simulink model "feedback_gravity_comp"  (R2019b)
settings: Solver=FixedStepAuto  StartTime=0.0  StopTime=inf  FixedStep=st  RelTol=1e-3
values from neighbouring files (symbols this model uses):
  p = pi    (= 3.14159265359)    [nominal_model.m]
libraries: arduinolib x18
settings Model: SILPILModeSetting=veronly  ExtModeTrigDuration=2  Creator=paniz  LastModifiedBy=paniz
settings OptimizationCC: EnhancedBackFolding=on  PassReuseOutputArgsAs=Individual arguments  ZeroExternalMemoryAtStartup=off  ZeroInternalMemoryAtStartup=off  MaxStackSize=64  OptimizeBlockOrder=speed  DifferentSizesBufferReuse=on  OptimizationCustomize=off  EfficientTunableParamExpr=on
settings DebuggingCC: ParameterTunabilityLossMsg=error  UnconnectedInputMsg=none  UnconnectedOutputMsg=none  UnconnectedLineMsg=none  SFMachineParentedDataDiag=error
settings HardwareCC: ProdBitPerInt=16  ProdBitPerPointer=16  ProdBitPerSizeT=16  ProdBitPerPtrDiffT=16  ProdLargestAtomicFloat=None  ProdWordSize=8  ProdHWDeviceType=Atmel->AVR
settings SFSimCC: MATLABDynamicMemAlloc=off
settings RTWCC: SystemTargetFile=ert.tlc  HardwareBoard=Arduino Mega 2560  TemplateMakefile=ert_default_tmf  Toolchain=Arduino AVR
settings CodeAppCC: ForceParamTrailComments=on  IgnoreCustomStorageClasses=off  OperatorAnnotations=on  SimulinkDataObjDesc=on  SFDataObjDesc=on  InsertBlockDesc=on
settings ERTTargetCC: SupportContinuousTime=on  SupportVariableSizeSignals=on  ExtMode=on  ExtModeTransport=3  ExtModeStaticAlloc=on  ExtModeStaticAllocSize=2048  ExtModeMexFile=ext_xcp  ExtModeMexArgs=0 5 921600 'C:\Users\paniz\myCodes\Using Arduino and Matlab\Codes\Simulink\3 Muscle with pressure regulator\untitled.elf' 3 1000  ExtModeIntrfLevel=Level2 - Open

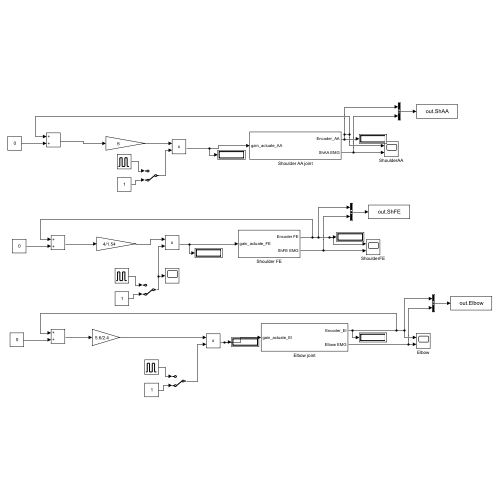
[thumbnail: Simulink's stored preview of the top-level diagram]
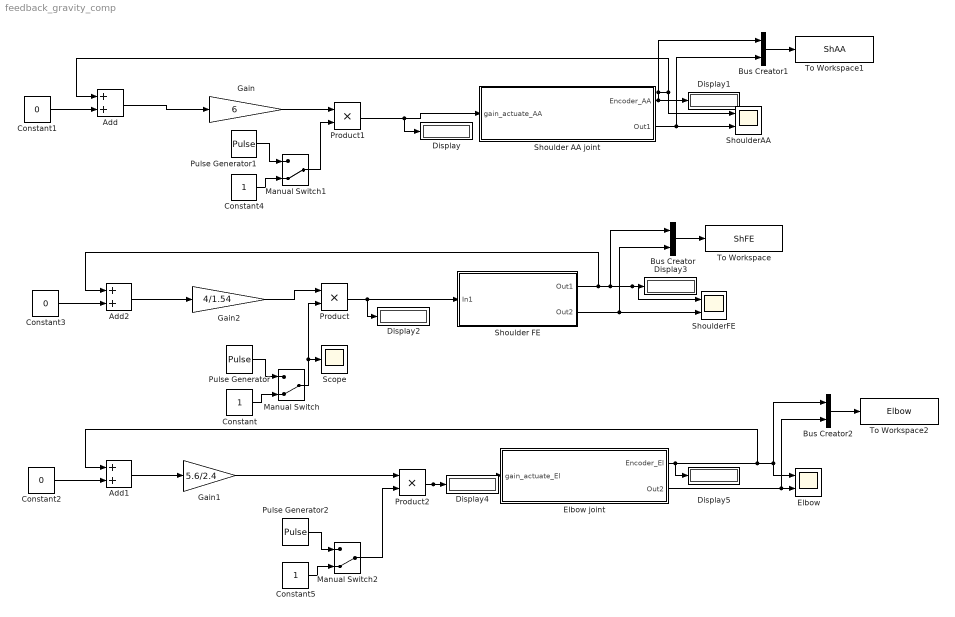
== system feedback_gravity_comp ==
  Add : Sum
  Add1 : Sum
  Add2 : Sum
  Bus Creator : BusCreator  Inputs=2
  Bus Creator1 : BusCreator  Inputs=2
  Bus Creator2 : BusCreator  Inputs=2
  Constant : Constant
  Constant1 : Constant  Value=0
  Constant2 : Constant  Value=0
  Constant3 : Constant  Value=0
  Constant4 : Constant
  Constant5 : Constant
  Display{,1..5} (6 alike) : Display
  Elbow : Scope  NumInputPorts=2
  Elbow joint : Subsystem
  Gain : Gain  Gain=6
  Gain1 : Gain  Gain=5.6/2.4
  Gain2 : Gain  Gain=4/1.54
  Manual Switch : ManualSwitch  CurrentSetting=0
  Manual Switch1 : ManualSwitch  CurrentSetting=0
  Manual Switch2 : ManualSwitch  CurrentSetting=0
  Product : Product
  Product1 : Product
  Product2 : Product
  Pulse Generator : DiscretePulseGenerator  PulseType=Time based  Period=7  PulseWidth=90
  Pulse Generator1 : DiscretePulseGenerator  PulseType=Time based  Period=7  PulseWidth=90
  Pulse Generator2 : DiscretePulseGenerator  PulseType=Time based  Period=7  PulseWidth=90
  Scope : Scope
  Shoulder AA joint : Subsystem
  Shoulder FE : Subsystem
  ShoulderAA : Scope  NumInputPorts=2
  ShoulderFE : Scope  NumInputPorts=2
  To Workspace : ToWorkspace  VariableName=ShFE  SampleTime=-1
  To Workspace1 : ToWorkspace  VariableName=ShAA  SampleTime=-1
  To Workspace2 : ToWorkspace  VariableName=Elbow  SampleTime=-1
  wires:
  Add/1 -> Gain/1
  Constant1/1 -> Add/2
  Constant2/1 -> Add1/2
  Add1/1 -> Gain1/1
  Shoulder AA joint/2(Out1) -> Bus Creator1/2, ShoulderAA/2
  Shoulder AA joint/1(Encoder_AA) -> Bus Creator1/1, ShoulderAA/1, Add/1, Display1/1
  Bus Creator1/1 -> To Workspace1/1
  Elbow joint/2(Out2) -> Bus Creator2/2, Elbow/2
  Elbow joint/1(Encoder_El) -> Elbow/1, Bus Creator2/1, Add1/1, Display5/1
  Bus Creator2/1 -> To Workspace2/1
  Manual Switch1/1 -> Product1/2
  Gain/1 -> Product1/1
  Product1/1 -> Display/1, Shoulder AA joint/1(gain_actuate_AA)
  Manual Switch2/1 -> Product2/2
  Gain1/1 -> Product2/1
  Constant4/1 -> Manual Switch1/2
  Pulse Generator1/1 -> Manual Switch1/1
  Constant5/1 -> Manual Switch2/2
  Pulse Generator2/1 -> Manual Switch2/1
  Manual Switch/1 -> Scope/1, Product/2
  Constant/1 -> Manual Switch/2
  Pulse Generator/1 -> Manual Switch/1
  Gain2/1 -> Product/1
  Product/1 -> Display2/1, Shoulder FE/1(In1)
  Shoulder FE/2(Out2) -> Bus Creator/2, ShoulderFE/2
  Add2/1 -> Gain2/1
  Constant3/1 -> Add2/2
  Shoulder FE/1(Out1) -> Add2/1, Bus Creator/1, ShoulderFE/1, Display3/1
  Bus Creator/1 -> To Workspace/1
  Product2/1 -> Elbow joint/1(gain_actuate_El), Display4/1

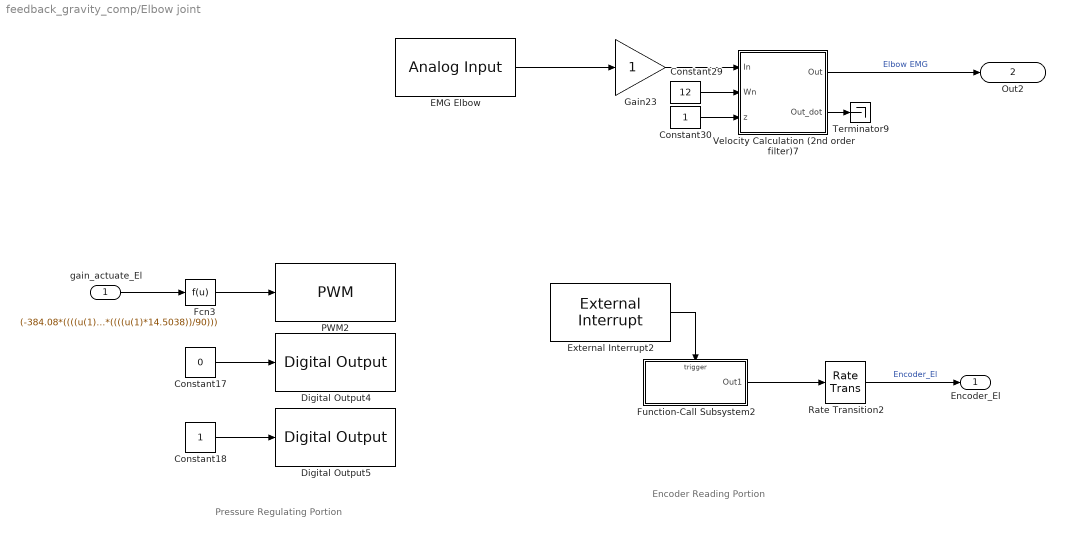
== system feedback_gravity_comp/Elbow joint ==
  note: Pressure Regulating Portion
  note: Encoder Reading Portion
  gain_actuate_El : Inport
  Constant17 : Constant  Value=0  SampleTime=-1
  Constant18 : Constant  SampleTime=-1
  Constant29 : Constant  Value=12
  Constant30 : Constant
  Digital Output4 : arduinolib/Digital Output  pinNumber=17  Direction=output  blockPlatform=arduino
  Digital Output5 : arduinolib/Digital Output  pinNumber=5  Direction=output  blockPlatform=arduino
  EMG Elbow : arduinolib/Analog Input  pinNumber=1  ReadResultsOnly=off  ConversionTriggerSource=Software  ExternalTriggerType=uint32( 0 )  OutputDataType=uint16  EnableConversionCompleteNotify=off  EnableOuputStatus=off  SampleTime=-1  blockPlatform=arduino
  External Interrupt2 : arduinolib/External Interrupt  Pin=3  PullUp=off  Mode=RISING  InterruptSimulationInput=off
      settings: SourceProductBaseCode=ARDUINO
  Fcn3 : Fcn  Expr=(-384.08*((((u(1)*14.5038))/90))^4 + 789.52*((((u(1)*14.5038))/90))^3 - 618.81*((((u(1)*14.5038))/90))^2 + 468.18*((((u(1)*14.5038))/90)))
  Function-Call Subsystem2 : Subsystem  TreatAsAtomicUnit=on
  Gain23 : Gain  OutDataTypeStr=double
  PWM2 : arduinolib/PWM  pinNumber=6  frequencyType=Specify  desiredFrequency=3921.16  achievableFrequency=3921.5686
  Rate Transition2 : RateTransition  Deterministic=off  OutPortSampleTimeOpt=Inherit
  Terminator9 : Terminator
  Velocity Calculation (2nd order filter)7 : Subsystem
  Encoder_El : Outport
  Out2 : Outport  Port=2
  wires:
  gain_actuate_El/1 -> Fcn3/1
  Fcn3/1 -> PWM2/1
  External Interrupt2/1 -> Function-Call Subsystem2/Trigger
  Function-Call Subsystem2/1(Out1) -> Rate Transition2/1
  Constant18/1 -> Digital Output5/1
  Constant17/1 -> Digital Output4/1
  Rate Transition2/1 -> Encoder_El/1  "Encoder_El"
  Velocity Calculation (2nd order filter)7/2(Out_dot) -> Terminator9/1
  EMG Elbow/1 -> Gain23/1
  Constant29/1 -> Velocity Calculation (2nd order filter)7/2(Wn)
  Gain23/1 -> Velocity Calculation (2nd order filter)7/1(In)
  Constant30/1 -> Velocity Calculation (2nd order filter)7/3(z)
  Velocity Calculation (2nd order filter)7/1(Out) -> Out2/1  "Elbow EMG"

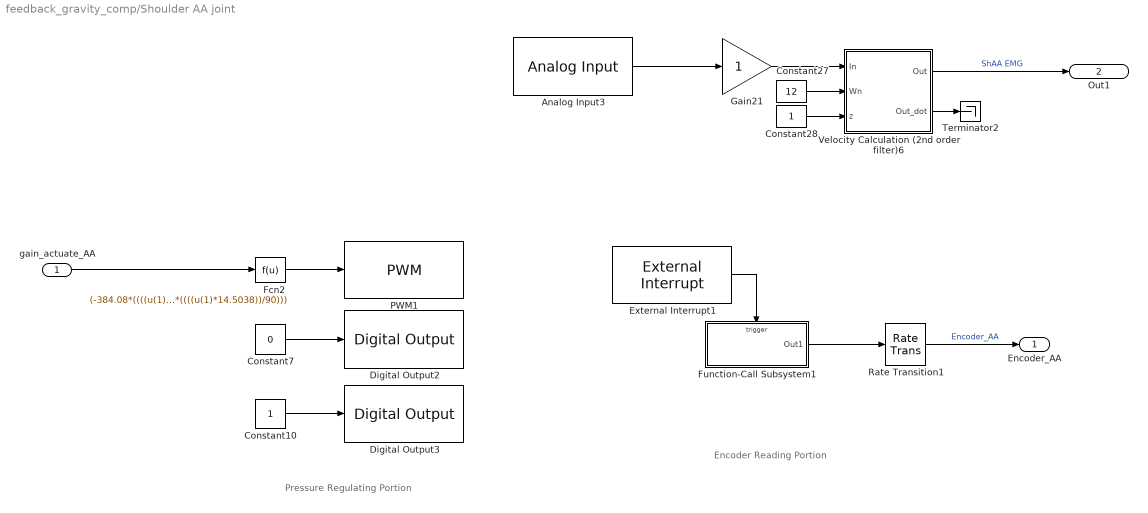
== system feedback_gravity_comp/Shoulder AA joint ==
  note: Pressure Regulating Portion
  note: Encoder Reading Portion
  gain_actuate_AA : Inport
  Analog Input3 : arduinolib/Analog Input  pinNumber=11  ReadResultsOnly=off  ConversionTriggerSource=Software  ExternalTriggerType=uint32( 0 )  OutputDataType=uint16  EnableConversionCompleteNotify=off  EnableOuputStatus=off  SampleTime=-1  blockPlatform=arduino
  Constant10 : Constant  SampleTime=-1
  Constant27 : Constant  Value=12
  Constant28 : Constant
  Constant7 : Constant  Value=0  SampleTime=-1
  Digital Output2 : arduinolib/Digital Output  pinNumber=52  Direction=output  blockPlatform=arduino
  Digital Output3 : arduinolib/Digital Output  pinNumber=53  Direction=output  blockPlatform=arduino
  External Interrupt1 : arduinolib/External Interrupt  Pin=20  PullUp=off  Mode=RISING  InterruptSimulationInput=off
      settings: SourceProductBaseCode=ARDUINO
  Fcn2 : Fcn  Expr=(-384.08*((((u(1)*14.5038))/90))^4 + 789.52*((((u(1)*14.5038))/90))^3 - 618.81*((((u(1)*14.5038))/90))^2 + 468.18*((((u(1)*14.5038))/90)))
  Function-Call Subsystem1 : Subsystem  TreatAsAtomicUnit=on
  Gain21 : Gain  OutDataTypeStr=double
  PWM1 : arduinolib/PWM  pinNumber=8  frequencyType=Specify  desiredFrequency=3921.16  achievableFrequency=3921.5686
  Rate Transition1 : RateTransition  Deterministic=off  OutPortSampleTimeOpt=Inherit
  Terminator2 : Terminator
  Velocity Calculation (2nd order filter)6 : Subsystem
  Encoder_AA : Outport
  Out1 : Outport  Port=2
  wires:
  Function-Call Subsystem1/1(Out1) -> Rate Transition1/1
  Constant7/1 -> Digital Output2/1
  Fcn2/1 -> PWM1/1
  Constant10/1 -> Digital Output3/1
  Rate Transition1/1 -> Encoder_AA/1  "Encoder_AA"
  External Interrupt1/1 -> Function-Call Subsystem1/Trigger
  gain_actuate_AA/1 -> Fcn2/1
  Velocity Calculation (2nd order filter)6/2(Out_dot) -> Terminator2/1
  Analog Input3/1 -> Gain21/1
  Constant27/1 -> Velocity Calculation (2nd order filter)6/2(Wn)
  Velocity Calculation (2nd order filter)6/1(Out) -> Out1/1  "ShAA EMG"
  Constant28/1 -> Velocity Calculation (2nd order filter)6/3(z)
  Gain21/1 -> Velocity Calculation (2nd order filter)6/1(In)

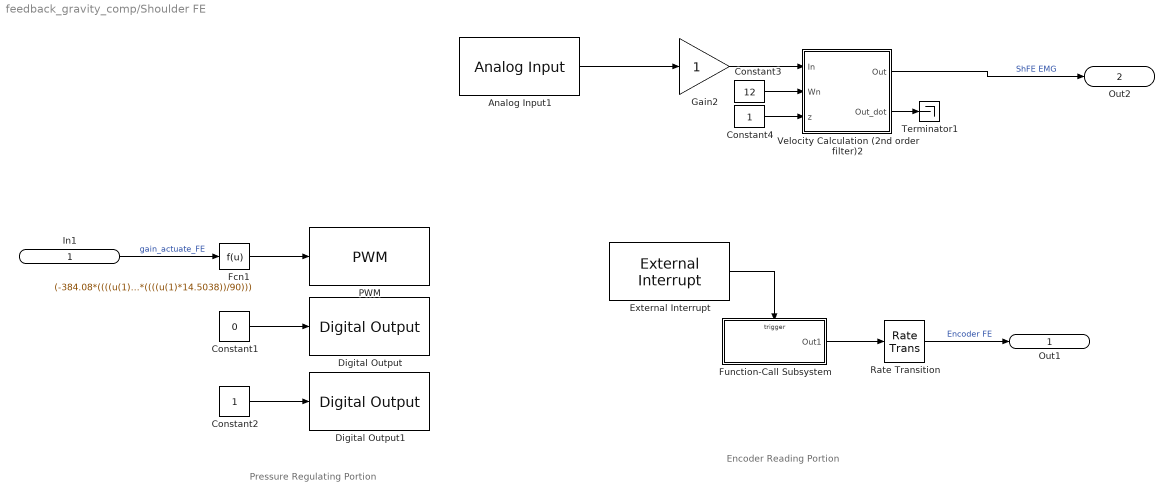
== system feedback_gravity_comp/Shoulder FE ==
  note: Encoder Reading Portion
  note: Pressure Regulating Portion
  In1 : Inport
  Analog Input1 : arduinolib/Analog Input  pinNumber=6  ReadResultsOnly=off  ConversionTriggerSource=Software  ExternalTriggerType=uint32( 0 )  OutputDataType=uint16  EnableConversionCompleteNotify=off  EnableOuputStatus=off  SampleTime=-1  blockPlatform=arduino
  Constant1 : Constant  Value=0  SampleTime=-1
  Constant2 : Constant  SampleTime=-1
  Constant3 : Constant  Value=12
  Constant4 : Constant
  Digital Output : arduinolib/Digital Output  pinNumber=44  Direction=output  blockPlatform=arduino
  Digital Output1 : arduinolib/Digital Output  pinNumber=45  Direction=output  blockPlatform=arduino
  External Interrupt : arduinolib/External Interrupt  Pin=18  PullUp=off  Mode=RISING  InterruptSimulationInput=off
      settings: SourceProductBaseCode=ARDUINO
  Fcn1 : Fcn  Expr=(-384.08*((((u(1)*14.5038))/90))^4 + 789.52*((((u(1)*14.5038))/90))^3 - 618.81*((((u(1)*14.5038))/90))^2 + 468.18*((((u(1)*14.5038))/90)))
  Function-Call Subsystem : Subsystem  TreatAsAtomicUnit=on
  Gain2 : Gain  OutDataTypeStr=double
  PWM : arduinolib/PWM  pinNumber=7  frequencyType=Specify  desiredFrequency=3921.16  achievableFrequency=3921.5686
  Rate Transition : RateTransition  Deterministic=off  OutPortSampleTimeOpt=Inherit
  Terminator1 : Terminator
  Velocity Calculation (2nd order filter)2 : Subsystem
  Out1 : Outport
  Out2 : Outport  Port=2
  wires:
  Constant1/1 -> Digital Output/1
  Constant2/1 -> Digital Output1/1
  Function-Call Subsystem/1(Out1) -> Rate Transition/1
  Fcn1/1 -> PWM/1
  External Interrupt/1 -> Function-Call Subsystem/Trigger
  In1/1 -> Fcn1/1  "gain_actuate_FE"
  Rate Transition/1 -> Out1/1  "Encoder FE"
  Velocity Calculation (2nd order filter)2/1(Out) -> Out2/1  "ShFE EMG"
  Analog Input1/1 -> Gain2/1
  Gain2/1 -> Velocity Calculation (2nd order filter)2/1(In)
  Constant3/1 -> Velocity Calculation (2nd order filter)2/2(Wn)
  Velocity Calculation (2nd order filter)2/2(Out_dot) -> Terminator1/1
  Constant4/1 -> Velocity Calculation (2nd order filter)2/3(z)

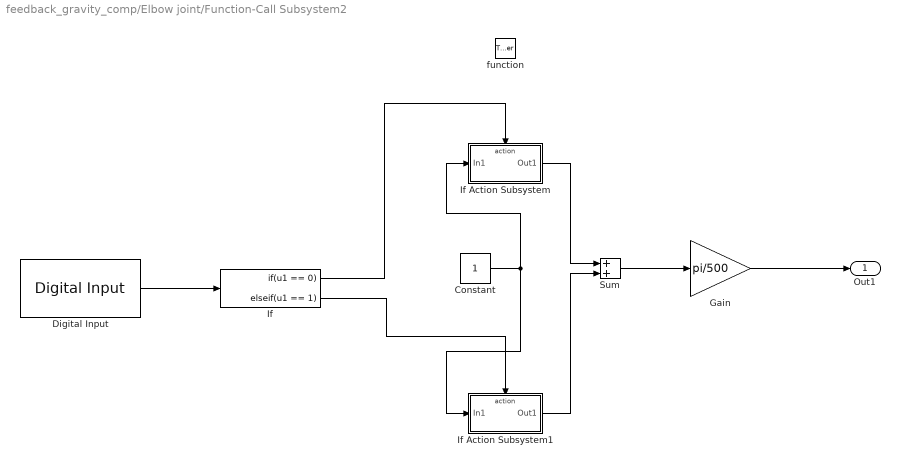
== system feedback_gravity_comp/Elbow joint/Function-Call Subsystem2 ==
  function : TriggerPort  TriggerType=function-call  VariantControl=Variant
  Constant : Constant
  Digital Input : arduinolib/Digital Input  pinNumber=2  mode=Default  Direction=input  SampleTime=-1  blockPlatform=arduino
  Gain : Gain  Gain=pi/500
  If : If  IfExpression=u1 == 0  ElseIfExpressions=u1 == 1  ShowElse=off
  If Action Subsystem : Subsystem  TreatAsAtomicUnit=on
  If Action Subsystem1 : Subsystem  TreatAsAtomicUnit=on
  Sum : Sum
  Out1 : Outport
  wires:
  If/1 -> If Action Subsystem/Action
  If/2 -> If Action Subsystem1/Action
  Constant/1 -> If Action Subsystem1/1(In1), If Action Subsystem/1(In1)
  If Action Subsystem/1(Out1) -> Sum/1
  Sum/1 -> Gain/1
  If Action Subsystem1/1(Out1) -> Sum/2
  Digital Input/1 -> If/1
  Gain/1 -> Out1/1

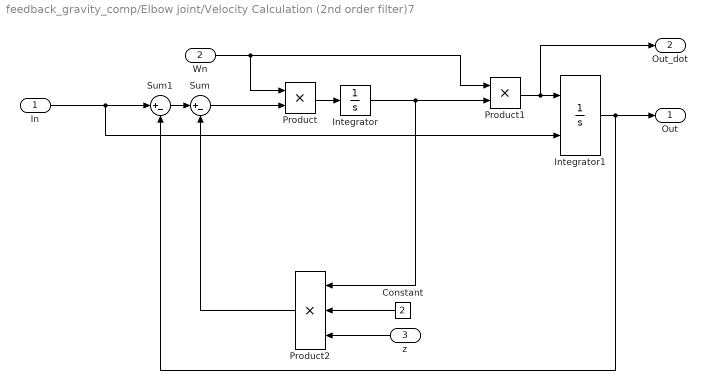
== system feedback_gravity_comp/Elbow joint/Velocity Calculation (2nd order filter)7 ==
  In : Inport
  Wn : Inport  Port=2
  z : Inport  Port=3
  Constant : Constant  Value=2
  Integrator : Integrator
  Integrator1 : Integrator  InitialConditionSource=external
  Product : Product  RndMeth=Zero
  Product1 : Product  RndMeth=Zero
  Product2 : Product  Inputs=3  RndMeth=Zero
  Sum : Sum  Inputs=|+-
  Sum1 : Sum  Inputs=|+-
  Out : Outport
  Out_dot : Outport  Port=2
  wires:
  Product/1 -> Integrator/1
  Sum/1 -> Product/2
  Wn/1 -> Product/1, Product1/1
  Product1/1 -> Integrator1/1, Out_dot/1
  Integrator/1 -> Product1/2, Product2/1
  Integrator1/1 -> Sum1/2, Out/1
  Sum1/1 -> Sum/1
  In/1 -> Sum1/1, Integrator1/2
  Product2/1 -> Sum/2
  z/1 -> Product2/3
  Constant/1 -> Product2/2

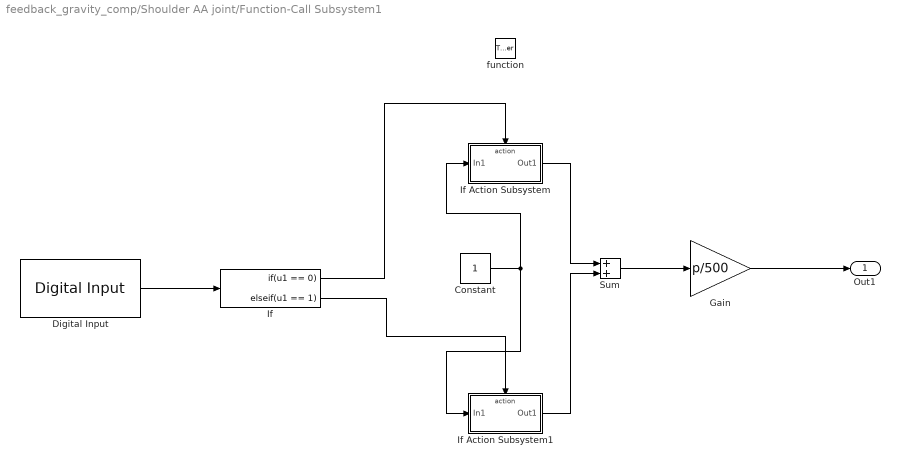
== system feedback_gravity_comp/Shoulder AA joint/Function-Call Subsystem1 ==
  function : TriggerPort  TriggerType=function-call  VariantControl=Variant
  Constant : Constant
  Digital Input : arduinolib/Digital Input  pinNumber=21  mode=Default  Direction=input  SampleTime=-1  blockPlatform=arduino
  Gain : Gain  Gain=p/500
  If : If  IfExpression=u1 == 0  ElseIfExpressions=u1 == 1  ShowElse=off
  If Action Subsystem : Subsystem  TreatAsAtomicUnit=on
  If Action Subsystem1 : Subsystem  TreatAsAtomicUnit=on
  Sum : Sum
  Out1 : Outport
  wires:
  If/1 -> If Action Subsystem/Action
  If/2 -> If Action Subsystem1/Action
  Constant/1 -> If Action Subsystem1/1(In1), If Action Subsystem/1(In1)
  If Action Subsystem/1(Out1) -> Sum/1
  Sum/1 -> Gain/1
  If Action Subsystem1/1(Out1) -> Sum/2
  Digital Input/1 -> If/1
  Gain/1 -> Out1/1

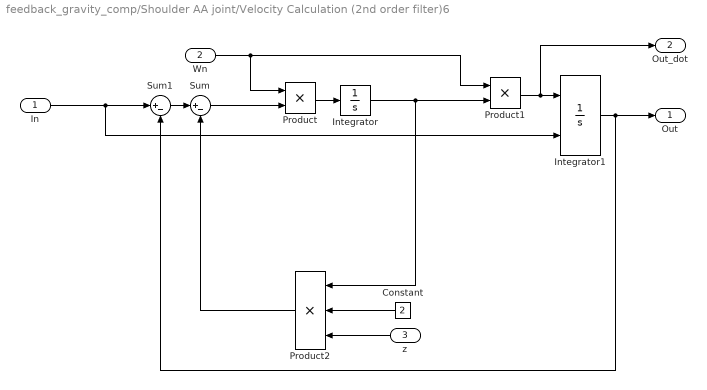
== system feedback_gravity_comp/Shoulder AA joint/Velocity Calculation (2nd order filter)6 ==
  In : Inport
  Wn : Inport  Port=2
  z : Inport  Port=3
  Constant : Constant  Value=2
  Integrator : Integrator
  Integrator1 : Integrator  InitialConditionSource=external
  Product : Product  RndMeth=Zero
  Product1 : Product  RndMeth=Zero
  Product2 : Product  Inputs=3  RndMeth=Zero
  Sum : Sum  Inputs=|+-
  Sum1 : Sum  Inputs=|+-
  Out : Outport
  Out_dot : Outport  Port=2
  wires:
  Product/1 -> Integrator/1
  Sum/1 -> Product/2
  Wn/1 -> Product/1, Product1/1
  Product1/1 -> Integrator1/1, Out_dot/1
  Integrator/1 -> Product1/2, Product2/1
  Integrator1/1 -> Sum1/2, Out/1
  Sum1/1 -> Sum/1
  In/1 -> Sum1/1, Integrator1/2
  Product2/1 -> Sum/2
  z/1 -> Product2/3
  Constant/1 -> Product2/2

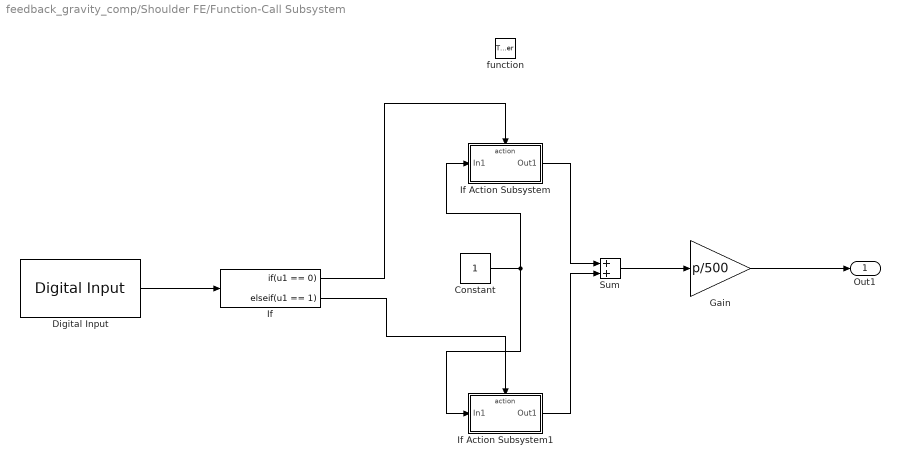
== system feedback_gravity_comp/Shoulder FE/Function-Call Subsystem ==
  function : TriggerPort  TriggerType=function-call  VariantControl=Variant
  Constant : Constant
  Digital Input : arduinolib/Digital Input  pinNumber=19  mode=Default  Direction=input  SampleTime=-1  blockPlatform=arduino
  Gain : Gain  Gain=p/500
  If : If  IfExpression=u1 == 0  ElseIfExpressions=u1 == 1  ShowElse=off
  If Action Subsystem : Subsystem  TreatAsAtomicUnit=on
  If Action Subsystem1 : Subsystem  TreatAsAtomicUnit=on
  Sum : Sum
  Out1 : Outport
  wires:
  If/1 -> If Action Subsystem/Action
  If/2 -> If Action Subsystem1/Action
  Constant/1 -> If Action Subsystem1/1(In1), If Action Subsystem/1(In1)
  If Action Subsystem/1(Out1) -> Sum/1
  Sum/1 -> Gain/1
  If Action Subsystem1/1(Out1) -> Sum/2
  Digital Input/1 -> If/1
  Gain/1 -> Out1/1

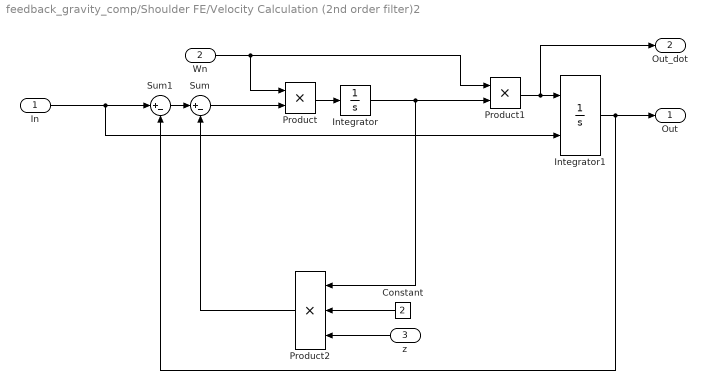
== system feedback_gravity_comp/Shoulder FE/Velocity Calculation (2nd order filter)2 ==
  In : Inport
  Wn : Inport  Port=2
  z : Inport  Port=3
  Constant : Constant  Value=2
  Integrator : Integrator
  Integrator1 : Integrator  InitialConditionSource=external
  Product : Product  RndMeth=Zero
  Product1 : Product  RndMeth=Zero
  Product2 : Product  Inputs=3  RndMeth=Zero
  Sum : Sum  Inputs=|+-
  Sum1 : Sum  Inputs=|+-
  Out : Outport
  Out_dot : Outport  Port=2
  wires:
  Product/1 -> Integrator/1
  Sum/1 -> Product/2
  Wn/1 -> Product/1, Product1/1
  Product1/1 -> Integrator1/1, Out_dot/1
  Integrator/1 -> Product1/2, Product2/1
  Integrator1/1 -> Sum1/2, Out/1
  Sum1/1 -> Sum/1
  In/1 -> Sum1/1, Integrator1/2
  Product2/1 -> Sum/2
  z/1 -> Product2/3
  Constant/1 -> Product2/2

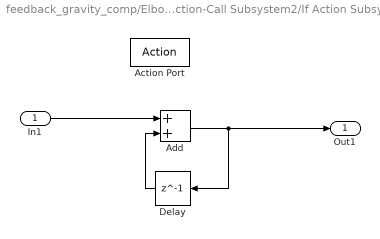
== system feedback_gravity_comp/Elbow joint/Function-Call Subsystem2/If Action Subsystem ==
  In1 : Inport
  Action Port : ActionPort  ActionPortLabel=if(u1 == 0)
  Add : Sum
  Delay : Delay  DelayLength=1
  Out1 : Outport
  wires:
  Add/1 -> Delay/1, Out1/1
  Delay/1 -> Add/2
  In1/1 -> Add/1

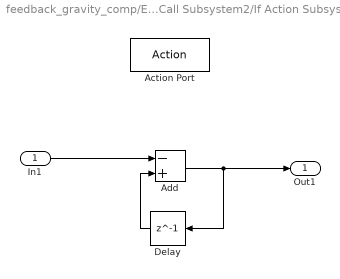
== system feedback_gravity_comp/Elbow joint/Function-Call Subsystem2/If Action Subsystem1 ==
  In1 : Inport
  Action Port : ActionPort  ActionPortLabel=elseif(u1 == 1)
  Add : Sum  Inputs=-+
  Delay : Delay  DelayLength=1
  Out1 : Outport
  wires:
  Delay/1 -> Add/2
  Add/1 -> Delay/1, Out1/1
  In1/1 -> Add/1

== system feedback_gravity_comp/Shoulder AA joint/Function-Call Subsystem1/If Action Subsystem ==
  In1 : Inport
  Action Port : ActionPort  ActionPortLabel=if(u1 == 0)
  Add : Sum
  Delay : Delay  DelayLength=1
  Out1 : Outport
  wires:
  Add/1 -> Delay/1, Out1/1
  Delay/1 -> Add/2
  In1/1 -> Add/1

== system feedback_gravity_comp/Shoulder AA joint/Function-Call Subsystem1/If Action Subsystem1 ==
  In1 : Inport
  Action Port : ActionPort  ActionPortLabel=elseif(u1 == 1)
  Add : Sum  Inputs=-+
  Delay : Delay  DelayLength=1
  Out1 : Outport
  wires:
  Delay/1 -> Add/2
  Add/1 -> Delay/1, Out1/1
  In1/1 -> Add/1

== system feedback_gravity_comp/Shoulder FE/Function-Call Subsystem/If Action Subsystem ==
  In1 : Inport
  Action Port : ActionPort  ActionPortLabel=if(u1 == 0)
  Add : Sum
  Delay : Delay  DelayLength=1
  Out1 : Outport
  wires:
  Add/1 -> Delay/1, Out1/1
  Delay/1 -> Add/2
  In1/1 -> Add/1

== system feedback_gravity_comp/Shoulder FE/Function-Call Subsystem/If Action Subsystem1 ==
  In1 : Inport
  Action Port : ActionPort  ActionPortLabel=elseif(u1 == 1)
  Add : Sum  Inputs=-+
  Delay : Delay  DelayLength=1
  Out1 : Outport
  wires:
  Delay/1 -> Add/2
  Add/1 -> Delay/1, Out1/1
  In1/1 -> Add/1
